simulink model "practice_final_part_5"  (R2015b)
settings: Solver=ode45  StartTime=0.0  StopTime=20  RelTol=1e-3
InitFcn:
  | param
undefined symbols (not defined in the file or in its folder): ctrl_loop, drawRodMass, P
libraries: simulink x1
settings Model: Creator=beard  LastModifiedBy=beard
settings DataIOCC: LimitDataPoints=off  SaveFormat=Array  SignalLoggingSaveFormat=ModelDataLogs
settings OptimizationCC: ExpressionDepthLimit=2147483647
settings DebuggingCC: UnderspecifiedInitializationDetection=Classic  MergeDetectMultiDrivingBlocksExec=none  FcnCallInpInsideContextMsg=UseLocalSettings  StateNameClashWarn=warning
settings HardwareCC: ProdBitPerPointer=32  ProdLargestAtomicFloat=None  ProdIntDivRoundTo=Undefined  ProdEndianess=Unspecified  ProdWordSize=32  ProdHWDeviceType=32-bit Generic
settings GRTTargetCC: GeneratePreprocessorConditionals=Disable all  CombineOutputUpdateFcns=off  GRTInterface=on
settings ConfigComp: CovModelRefEnable=Off

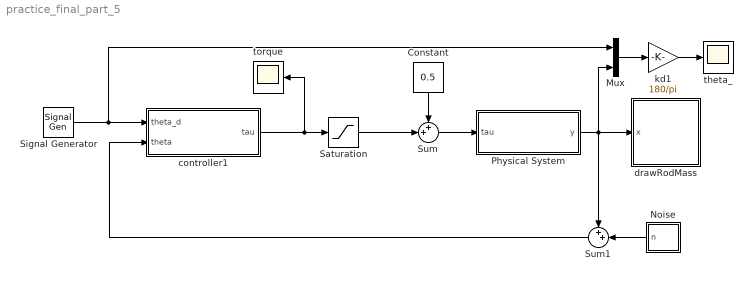
== system practice_final_part_5 ==
  Constant : Constant  Value=0.5
  Mux : Mux  Inputs=2
  Noise : Subsystem
  Physical System : Subsystem
  Saturation : Saturate  UpperLimit=P.tau_max  LowerLimit=-P.tau_max
  Signal Generator : SignalGenerator  WaveForm=square  Amplitude=10*pi/180  Frequency=.1
  Sum : Sum  Inputs=++|
  Sum1 : Sum  Inputs=++|
  controller1 : Subsystem
  drawRodMass : Subsystem
      mask init:
      | % drawing parameters
      | L = 1;
      | w = 0.01;
      | R = 0.1;
      | H = 1;
      mask Display: image(imread('tv.jpg'))
  kd1 : Gain  Gain=180/pi
  theta_ : Scope
  torque : Scope
  wires:
  Mux/1 -> kd1/1
  kd1/1 -> theta_/1
  Signal Generator/1 -> controller1/1(theta_d), Mux/1
  Physical System/1(y) -> drawRodMass/1(x), Mux/2, Sum1/1
  Saturation/1 -> Sum/2
  Sum/1 -> Physical System/1(tau)
  Constant/1 -> Sum/1
  Sum1/1 -> controller1/2(theta)
  Noise/1(n) -> Sum1/2
  controller1/1(tau) -> torque/1, Saturation/1

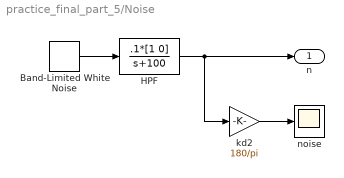
== system practice_final_part_5/Noise ==
  Band-Limited White Noise : simulink/Sources/Band-Limited White Noise  Cov=[0.001]  Ts=0.1  seed=[23341]
  HPF : TransferFcn  Numerator=.1*[1 0]  Denominator=[1 100]
  kd2 : Gain  Gain=180/pi
  noise : Scope
  n : Outport
  wires:
  Band-Limited White Noise/1 -> HPF/1
  kd2/1 -> noise/1
  HPF/1 -> kd2/1, n/1

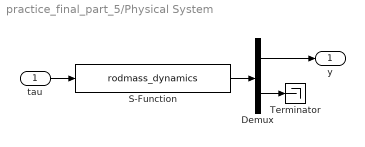
== system practice_final_part_5/Physical System ==
  tau : Inport
  Demux : Demux  Outputs=[1;2]
  S-Function : S-Function  FunctionName=rodmass_dynamics  SFunctionDeploymentMode=off  EnableBusSupport=off
  Terminator : Terminator
  y : Outport
  wires:
  tau/1 -> S-Function/1
  S-Function/1 -> Demux/1
  Demux/2 -> Terminator/1
  Demux/1 -> y/1

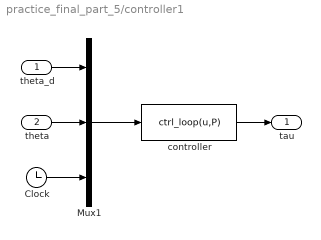
== system practice_final_part_5/controller1 ==
  theta_d : Inport
  theta : Inport  Port=2
  Clock : Clock
  Mux1 : Mux  Inputs=3
  controller : MATLABFcn  MATLABFcn=ctrl_loop(u,P)  OutputDimensions=1  SampleTime=P.Ts
  tau : Outport
  wires:
  Clock/1 -> Mux1/3
  controller/1 -> tau/1
  theta/1 -> Mux1/2
  theta_d/1 -> Mux1/1
  Mux1/1 -> controller/1

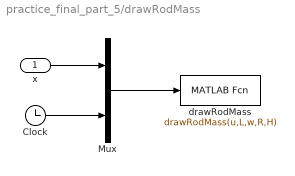
== system practice_final_part_5/drawRodMass ==
  x : Inport
  Clock : Clock
  Mux : Mux  Inputs=2
  drawRodMass : MATLABFcn  MATLABFcn=drawRodMass(u,L,w,R,H)  OutputDimensions=0  SampleTime=0.1
  wires:
  Clock/1 -> Mux/2
  x/1 -> Mux/1
  Mux/1 -> drawRodMass/1
